simulink model "model_wahadla"  (R2023a)
settings: Solver=ode45  StartTime=0.0  StopTime=end_time  FixedStep=dt  MaxStep=0.001  RelTol=1e-3
undefined symbols (not defined in the file or in its folder): A, B, C, D, IC
settings Model: Creator=Adam  LastModifiedBy=domrazek
settings SolverCC: AlgebraicLoopSolver=TrustRegion
settings DataIOCC: ExternalInput=ind  LoadExternalInput=on  SignalLogging=off  DSMLogging=off  OutputSaveName=out  ReturnWorkspaceOutputsName=sout
settings OptimizationCC: SimCompilerOptimization=on  AccelVerboseBuild=on
settings DebuggingCC: AlgebraicLoopMsg=none  UnconnectedInputMsg=warning  UnconnectedOutputMsg=warning  UnconnectedLineMsg=warning
settings ModelReferenceCC: EnableRefExpFcnMdlSchedulingChecks=on
settings RTWCC: DLArmComputeVersion=19.05

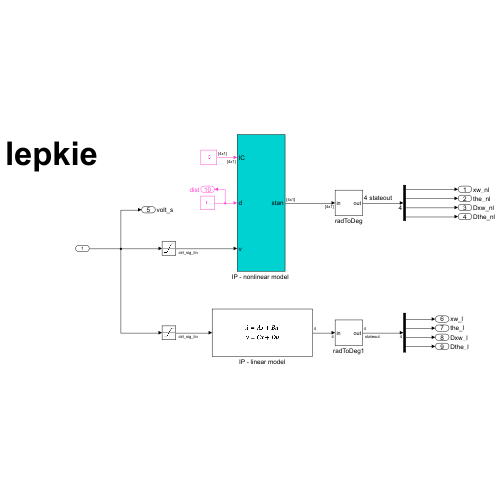
[thumbnail: Simulink's stored preview of the top-level diagram]
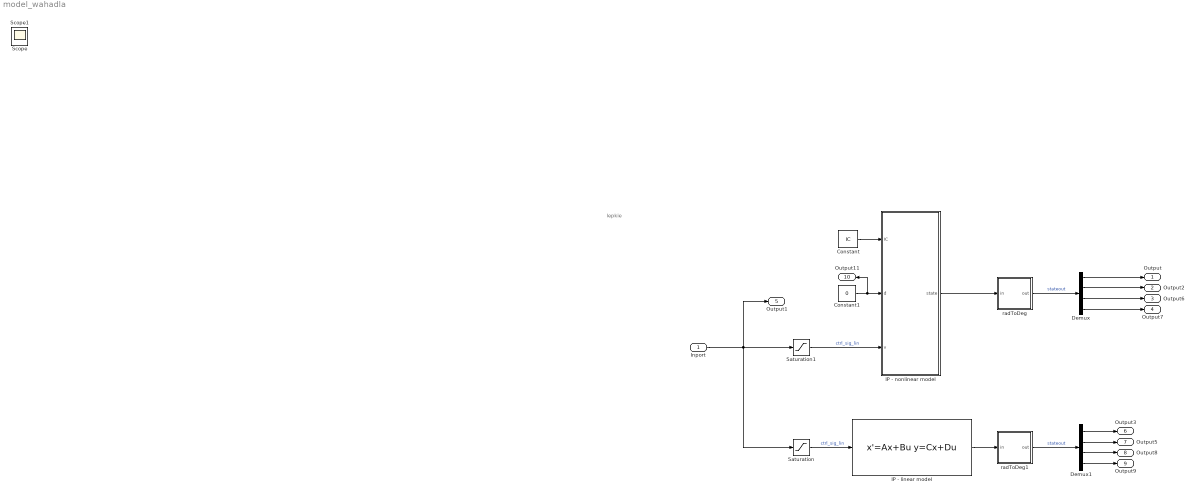
== system model_wahadla ==
  note: lepkie
  Inport : Inport
  Constant : Constant  Value=IC  VectorParams1D=off
  Constant1 : Constant  Value=0
  Demux : Demux
  Demux1 : Demux
  IP - linear model : StateSpace  A=A  B=B  C=C  D=D  InitialCondition=IC
  "IP - nonlinear model " : Subsystem  Description=Nonlinear model of inverted pendulum
      mask Display:
      | port_label('output', 1, 'stan');
      | port_label('input', 1, 'IC');
      | port_label('input', 2, 'd');
      | port_label('input', 3, 'v');
  Saturation : Saturate  UpperLimit=12  LowerLimit=-12
  Saturation1 : Saturate  UpperLimit=12  LowerLimit=-12
  radToDeg : Subsystem
  radToDeg1 : Subsystem
  Output : Outport  SignalName=xw_nl
  Output2 : Outport  Port=2  SignalName=the_nl
  Output6 : Outport  Port=3  SignalName=Dxw_nl
  Output7 : Outport  Port=4  SignalName=Dthe_nl
  Output1 : Outport  Port=5  SignalName=volt_s
  Output3 : Outport  Port=6  SignalName=xw_l
  Output5 : Outport  Port=7  SignalName=the_l
  Output8 : Outport  Port=8  SignalName=Dxw_l
  Output9 : Outport  Port=9  SignalName=Dthe_l
  Output11 : Outport  Port=10  SignalName=dist
  Scope : Scope
  Scope1 : Scope
  wires:
  "IP - nonlinear model "/1(state) -> radToDeg/1(in)
  Constant/1 -> "IP - nonlinear model "/1(IC)
  Constant1/1 -> "IP - nonlinear model "/2(d), Output11/1
  radToDeg/1(out) -> Demux/1  "stateout"
  Demux/1 -> Output/1
  Demux/2 -> Output2/1
  Demux/3 -> Output6/1
  Demux/4 -> Output7/1
  Saturation/1 -> IP - linear model/1  "ctrl_sig_lin"
  IP - linear model/1 -> radToDeg1/1(in)
  Demux1/1 -> Output3/1
  Demux1/2 -> Output5/1
  Demux1/3 -> Output8/1
  Demux1/4 -> Output9/1
  radToDeg1/1(out) -> Demux1/1  "stateout"
  Inport/1 -> Saturation1/1, Output1/1, Saturation/1
  Saturation1/1 -> "IP - nonlinear model "/3(v)  "ctrl_sig_lin"

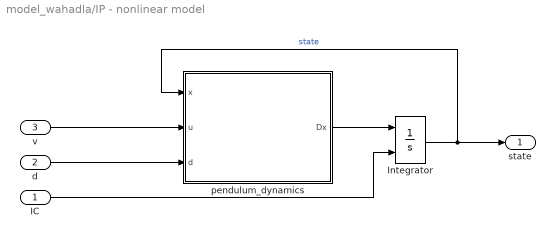
== system model_wahadla/IP - nonlinear model  ==
  IC : Inport
  d : Inport  Port=2
  v : Inport  Port=3
  Integrator : Integrator  InitialConditionSource=external
  pendulum_dynamics : MATLAB Function  TreatAsAtomicUnit=on
  state : Outport
  wires:
  Integrator/1 -> state/1, pendulum_dynamics/1(x)  "state"
  v/1 -> pendulum_dynamics/2(u)
  pendulum_dynamics/1(Dx) -> Integrator/1
  IC/1 -> Integrator/2
  d/1 -> pendulum_dynamics/3(d)

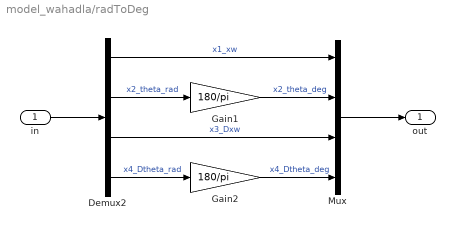
== system model_wahadla/radToDeg ==
  in : Inport
  Demux2 : Demux
  Gain1 : Gain  Gain=180/pi
  Gain2 : Gain  Gain=180/pi
  Mux : Mux
  out : Outport
  wires:
  Demux2/1 -> Mux/1  "x1_xw"
  Gain1/1 -> Mux/2  "x2_theta_deg"
  Gain2/1 -> Mux/4  "x4_Dtheta_deg"
  Demux2/2 -> Gain1/1  "x2_theta_rad"
  in/1 -> Demux2/1
  Demux2/3 -> Mux/3  "x3_Dxw"
  Demux2/4 -> Gain2/1  "x4_Dtheta_rad"
  Mux/1 -> out/1

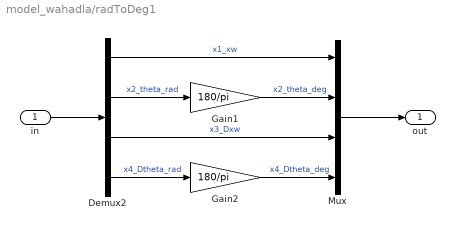
== system model_wahadla/radToDeg1 ==
  in : Inport
  Demux2 : Demux
  Gain1 : Gain  Gain=180/pi
  Gain2 : Gain  Gain=180/pi
  Mux : Mux
  out : Outport
  wires:
  Demux2/1 -> Mux/1  "x1_xw"
  Gain1/1 -> Mux/2  "x2_theta_deg"
  Gain2/1 -> Mux/4  "x4_Dtheta_deg"
  Demux2/2 -> Gain1/1  "x2_theta_rad"
  in/1 -> Demux2/1
  Demux2/3 -> Mux/3  "x3_Dxw"
  Demux2/4 -> Gain2/1  "x4_Dtheta_rad"
  Mux/1 -> out/1

== matlab function model_wahadla/IP - nonlinear model /pendulum_dynamics ==
  data: x input; u input; d input; Dx output; params_lepkie parameter
function Dx = dynamika_wahadla(x, u, d, params_lepkie)
% x : stan
% u : input - napięcie
%
% params scope: "parameters"
%

% State, function input: x = [x Dx theta Dtheta]'
x1 = x(1);
x2 = x(2); 
x3 = x(3);
x4 = x(4);

% if (x1 >= 0.47)
%    x1 = 0.47;
%    x2 = 0;
% elseif (x1 <= 0)
%    x1 = 0;
%    x2 = 0;
% end

params_lepkie = num2cell(params_lepkie);
[M, mc, mp, Lp, Lc, g, b, gamma, mr, Mt, L, Jcm, Jt, alpha, beta] = params_lepkie{:};

% Equations for pendulum dynamics
Ff = b*x3;
Fi = alpha*u - beta*x3;
A = d*cos(x2) - Ff + L*mr*x4^2*sin(x2) + Fi;
B = d*Lc + L*g*mr*sin(x2) - gamma*x4;
DEN = Jt*Mt - (L*mr*cos(x2))^2;

ddt_x1 = x3;
ddt_x2 = x4;
ddt_x3 = (Jt*A - L*mr*cos(x2)*B) / DEN;
ddt_x4 = (Mt*B - L*mr*cos(x2)*A) / DEN;

% output (wektor kolumnowy)
Dx = [ddt_x1 ddt_x2 ddt_x3 ddt_x4]';

end
